simulink model "IO601canJ1939loopback"  (R2012b)
settings: Solver=FixedStepDiscrete  StartTime=0.0  StopTime=inf  RelTol=1e-3
libraries: xpcJ1939lib x7, speedgoatlib_IO601 x3, simulink x3, xpclib x2
Description:
  | 7.14.0.739 (R2012a)
settings Model: BufferReuse=off  Creator=cedric  LastModifiedBy=lab3
settings SolverCC: EnableConcurrentExecution=on
settings DataIOCC: SignalLoggingSaveFormat=ModelDataLogs
settings OptimizationCC: BlockReduction=off  OptimizeBlockIOStorage=off  BufferReuse=off  ExpressionFolding=off  LocalBlockOutputs=off
settings DebuggingCC: FcnCallInpInsideContextMsg=UseLocalSettings
settings HardwareCC: ProdIntDivRoundTo=Zero  ProdEndianess=LittleEndian  ProdHWDeviceType=Generic->32-bit x86 compatible
settings RTWCC: SystemTargetFile=xpctarget.tlc  TemplateMakefile=xpc_default_tmf  Description=Simulink Real-Time  RTWVerbose=off  ProcessScript=xpctarget_make_rtw_hook  RTWCompilerOptimization=On
settings CodeAppCC: CustomSymbolStrType=$N$R$M_T
settings xpcTargetCC: TargetFcnLib=ansi_tfl_table_tmw.mat  CodeReplacementLibrary=XPC_BLAS  ParMdlRefBuildCompliant=on  ConcurrentExecutionCompliant=on  CombineSignalStateStructs=off  GRTInterface=on  GenerateAllocFcn=off  xPCTaskExecutionProfile=off  xPCRL32EventNumber=5000  xPCLoadParamSetFile=off  xPCConcurrentTasks=off  xPCEnableSFAnimation=off

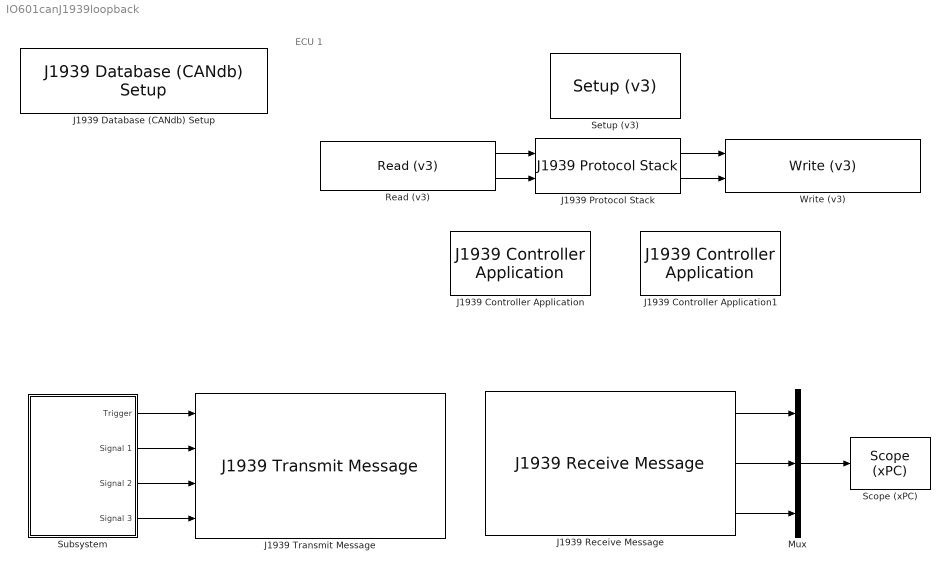
== system IO601canJ1939loopback ==
  note: ECU 1
  J1939 Controller Application : xpcJ1939lib/J1939 Controller Application  Priority=-1  stack_id=1  ca_id=1  node_addr=1  status=off  naddr_out=off  id_no=1  man_code=0  ecu_ins=0  func_ins=0  func=0  res=0  veh_sys=0  veh_sys_ins=0  ind_grp=0  aac=on  name_array=1|0|0|0|0|0|0|0|0|1
  J1939 Controller Application1 : xpcJ1939lib/J1939 Controller Application  Priority=-1  stack_id=1  ca_id=2  node_addr=2  status=off  naddr_out=off  id_no=2  man_code=0  ecu_ins=0  func_ins=0  func=0  res=0  veh_sys=0  veh_sys_ins=0  ind_grp=0  aac=on  name_array=2|0|0|0|0|0|0|0|0|1
  J1939 Database (CANdb) Setup : xpcJ1939lib/J1939 Database (CANdb) Setup  j1939dbcfilename=IO601canJ1939_db.dbc  dbcformat=1  updateBlock=1  ShowInLibBrowser=0
  J1939 Protocol Stack : xpcJ1939lib/J1939 Protocol Stack  Priority=-2  stack_id=1  max_rx=5  max_tx=20  tp_enabled=on  max_tp_sessions=10  ac_enabled=on  sample_rate=-1
  J1939 Receive Message : xpcJ1939lib/J1939 Receive Message  Priority=0  pgnindex=65210  stack_id=1  ca_id=2  node_addr=2  sourceAddress=255  destinationType=1  rx_status=0  updateBlock=0
  J1939 Transmit Message : xpcJ1939lib/J1939 Transmit Message  Priority=0  input_type=1  candb_filename=0  candb_format=1  pgnindex=65210  acronym=0  stack_id=1  ca_id=1  node_addr=1  messagePriority=0  destinationAddress=255  updateBlock=0
  Mux : Mux  Inputs=3
  Read (v3) : speedgoatlib_IO601/Read (v3)  id=1  outputFormat=Vector of CAN_MESSAGE  port1=off  port2=on  depth1=4  depth2=4  sampletime=0.001  pciSlot=-1
  Scope (xPC) : xpclib/Misc./Scope (xPC)   scopeno=1  scopetype=Target  autostart=on  viewmode=Numerical  formatstr='Signal 1: %10.3f,Signal 2: %10.3f,Signal 3: %10.3f'  grid=on  ylimits=[0,0]  nosamples=5  noprepostsamples=0  interleave=1  triggermode=FreeRun  triggersignal=1  trigsignalfromport=off  triggerlevel=0.0  triggerslope=Either  triggerscope=1  triggersample=0  filename=data.dat  mode=Lazy  writesize=512  autorestart=off  dynamicfilemode=off  maxwritefilesize=512*1024^2
  Setup (v3) : speedgoatlib_IO601/Setup (v3)  id=1  can1enable=on  can1bus=Highspeed  can1Baudrate=1 MBaud  can1UserBR=[1,1,5,2]  stdAcc1=[0,0,0,0]  extAcc1=[0,0,0,0]  can2enable=on  can2bus=Highspeed  can2Baudrate=1 MBaud  can2UserBR=[1,1,5,2]  stdAcc2=[0,0,0,0]  extAcc2=[0,0,0,0]  pciSlot=-1
  Subsystem : Subsystem
  Write (v3) : speedgoatlib_IO601/Write (v3)  Priority=1  id=1  sampletime=0.001  pciSlot=-1  inputType=CAN_MESSAGE plus count  port=1  maxMsg=20  status=off  init=[]  term=[]
  wires:
  Subsystem/4(Signal 3) -> J1939 Transmit Message/4
  Mux/1 -> Scope (xPC)/1
  Subsystem/2(Signal 1) -> J1939 Transmit Message/2
  Subsystem/3(Signal 2) -> J1939 Transmit Message/3
  J1939 Receive Message/1 -> Mux/1
  J1939 Receive Message/2 -> Mux/2
  Read (v3)/1 -> J1939 Protocol Stack/1
  J1939 Receive Message/3 -> Mux/3
  J1939 Protocol Stack/1 -> Write (v3)/1
  Subsystem/1(Trigger) -> J1939 Transmit Message/1
  J1939 Protocol Stack/2 -> Write (v3)/2
  Read (v3)/2 -> J1939 Protocol Stack/2

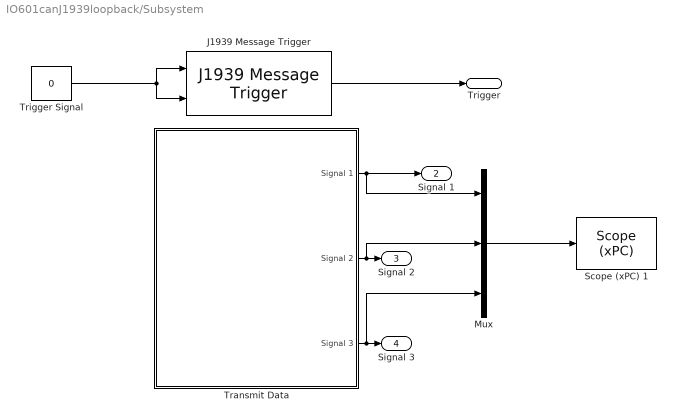
== system IO601canJ1939loopback/Subsystem ==
  J1939 Message Trigger : xpcJ1939lib/J1939 Message Trigger  repeatOnInterval=on  repetitionInterval=10  sendOnChange=on  changeThreshold=10  minChangeInterval=0
  Mux : Mux  Inputs=3
  Scope (xPC) 1 : xpclib/Misc./Scope (xPC)   scopeno=3  scopetype=Target  autostart=on  viewmode=Numerical  formatstr='Signal 1: %10.3f,Signal 2: %10.3f,Signal 3: %10.3f'  grid=on  ylimits=[0,0]  nosamples=5  noprepostsamples=0  interleave=1  triggermode=FreeRun  triggersignal=1  trigsignalfromport=off  triggerlevel=0.0  triggerslope=Either  triggerscope=1  triggersample=0  filename=data.dat  mode=Lazy  writesize=512  autorestart=off  dynamicfilemode=off  maxwritefilesize=512*1024^2
  Transmit Data : Subsystem
  Trigger Signal : Constant  Value=0
  Trigger : Outport
  Signal 1 : Outport  Port=2
  Signal 2 : Outport  Port=3
  Signal 3 : Outport  Port=4
  wires:
  J1939 Message Trigger/1 -> Trigger/1
  Trigger Signal/1 -> J1939 Message Trigger/1, J1939 Message Trigger/2
  Transmit Data/1(Signal 1) -> Mux/1, Signal 1/1
  Transmit Data/2(Signal 2) -> Mux/2, Signal 2/1
  Transmit Data/3(Signal 3) -> Mux/3, Signal 3/1
  Mux/1 -> Scope (xPC) 1/1

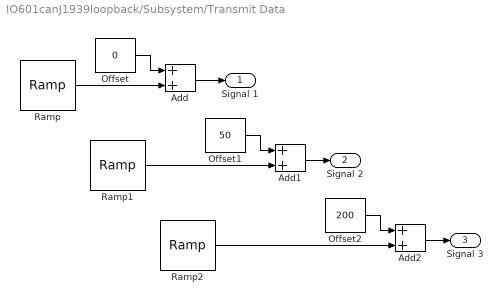
== system IO601canJ1939loopback/Subsystem/Transmit Data ==
  Add : Sum
  Add1 : Sum
  Add2 : Sum
  Offset : Constant  Value=0
  Offset1 : Constant  Value=50
  Offset2 : Constant  Value=200
  Ramp : simulink/Sources/Ramp  slope=0.125  start=0  X0=0
  Ramp1 : simulink/Sources/Ramp  slope=0.125  start=0  X0=0
  Ramp2 : simulink/Sources/Ramp  slope=0.125  start=0  X0=0
  Signal 1 : Outport
  Signal 2 : Outport  Port=2
  Signal 3 : Outport  Port=3
  wires:
  Offset/1 -> Add/1
  Ramp/1 -> Add/2
  Offset1/1 -> Add1/1
  Ramp1/1 -> Add1/2
  Ramp2/1 -> Add2/2
  Offset2/1 -> Add2/1
  Add/1 -> Signal 1/1
  Add1/1 -> Signal 2/1
  Add2/1 -> Signal 3/1
